simulink model "RHex1v3_Z_0v1b_PID"  (Simulink 7.9)
settings: Solver=ode23t  StartTime=0.0  StopTime=tp*3  MaxStep=0.005  RelTol=1e-3
values from neighbouring files (symbols this model uses):
  C = 100    [groundContact_init.m]
  Gvis = 0.01    [groundContact_init.m]
  K = x(5)    [PSO.m]    (also in PSO2_Kconst.m = 865; PSO3_PID.m = 525.4; bClockGen1v3_fin_acc.m = 1000; groundContact_init.m = 1000)
  kd = x(3)    [PSO3_PID.m]
  ki = x(2)    [PSO3_PID.m]
  kn = x(4)    [PSO3_PID.m]
  kp = x(1)    [PSO3_PID.m]
  m = 2    [PSO.m]    (also in PSO2_Kconst.m)
  nux = 1    [groundContact_init.m]
  nuy = 1    [groundContact_init.m]
  psziL = [psziL 360+psziL 720+psziL 1080+psziL]    [bClocGen1v3_fun.m]    (also in bClockGen1v3_fin_acc.m)
  psziR = [psziR 360+psziR 720+psziR 1080+psziR]    [bClocGen1v3_fun.m]    (also in bClockGen1v3_fin_acc.m)
  tp = x(1)    [PSO.m]    (also in PSO2_Kconst.m; PSO3_PID.m = 1.6; bClockGen1v3_fin_acc.m = 3)
undefined symbols (not defined in the file or in its folder): Body, deg, lab_rogz1v1, RHex1v3, RHex1v3_Z, RootPart, s
libraries: mblibv1 x64, Ervin x12, simulink x8
(part 1 of 2)
settings Model: Creator=Cloud  LastModifiedBy=Cloud
settings SimMechanicsCC: VisOnUpdateDiagram=on  VisDuringSimulation=on
settings ConfigurationSet: Description=SimMechanics 2G

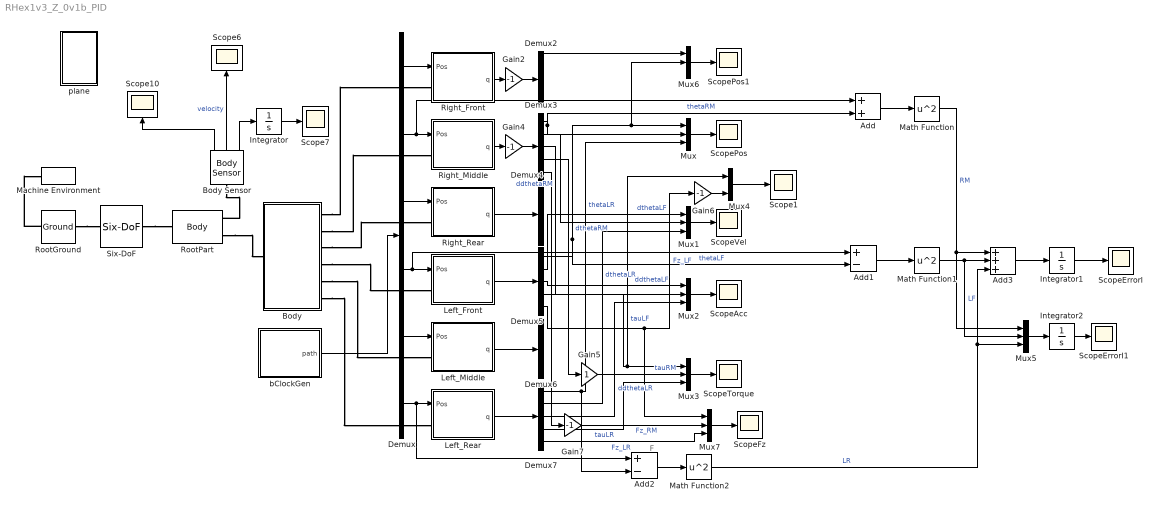
== system RHex1v3_Z_0v1b_PID ==
  note: F
  Add : Sum
  Add1 : Sum  Inputs=+-
  Add2 : Sum  Inputs=+-
  Add3 : Sum  Inputs=+++
  Body : Subsystem
  Body Sensor : mblibv1/Sensors &  Actuators/Body Sensor  UpdateFromCAD=off  PhysicalDomain=Mechanical  PortType=blob  Muxed=off  Pose=off  Angle=on  AngleUnits=deg  ArcVelocity=on  ArcVelocityUnits=deg/s  ArcAcceleration=off  ArcAccelerationUnits=deg/s^2  CoordPosition=on  CoordPositionUnits=mm  Velocity=on  VelocityUnits=m/s  Acceleration=off  AccelerationUnits=m/s^2  Quaternion=on  QuaternionDT=off  QuaternionDDT=off  QuaternionUnits=off  OutputVector=[1]  ActiveIO=on  Width=9  DialogClass=MechanicalSensorBlock  ReferenceFrame=Absolute (World)
  Demux : Demux  Outputs=6
  Demux{2..7} (6 alike) : Demux  Outputs=5
  Gain{2,4,6..7} (4 alike) : Gain  Gain=-1
  Gain5 : Gain
  Integrator : Integrator
  Integrator1 : Integrator
  Integrator2 : Integrator
  Left_Front : Subsystem
  Left_Middle : Subsystem
  Left_Rear : Subsystem
  Machine Environment : mblibv1/Bodies/Machine Environment  PortType=env  PhysicalDomain=Mechanical  DialogTemplateClass=MECH.MachineEnvironment  SyncWhenCopied=off  Gravity=[0 0 -9.81]  GravityUnits=m/s^2  GravityAsSignal=off  Dimensionality=Auto-detect  AnalysisType=Forward dynamics  LinearAssemblyTolerance=1e-3  LinearAssemblyToleranceUnits=m  AngularAssemblyTolerance=1e-3  AngularAssemblyToleranceUnits=rad  ConstraintSolverType=Stabilizing  ConstraintRelTolerance=1e-4  ConstraintAbsTolerance=1e-4  UseRobustSingularityHandling=off  RedundancyAnalysisToleranceType=Automatically select tolerance  RedundancyAnalysisTolerance=1e-14  StatePerturbationType=Fixed  PerturbationSize=1e-5  VisualizeMachine=on  BodyVisualizationType=Use model default body geometries  BodyColorSelMode=Use model default  DefaultBodyColor=[1 0 0]
  Math Function : Math  Operator=square  SaturateOnIntegerOverflow=on
  Math Function1 : Math  Operator=square  SaturateOnIntegerOverflow=on
  Math Function2 : Math  Operator=square  SaturateOnIntegerOverflow=on
  Mux{,1..3,5..7} (7 alike) : Mux  Inputs=3
  Mux4 : Mux  Inputs=2
  Right_Front : Subsystem
  Right_Middle : Subsystem
  Right_Rear : Subsystem
  RootGround : mblibv1/Bodies/Ground  UpdateFromCAD=on  PMImportedID=RootGround  LeftPortType=env  RightPortType=workingframe  PhysicalDomain=Mechanical  DialogClass=GroundBlock  CoordPosition=[-0.165584,-0.156961,0.0648014]  CoordPositionUnits=m  StateVectorMgrId=0  MachineId=[1 0]  ShowEnvPort=on
  RootPart : mblibv1/Bodies/Body  LConnTagsString=CS3  RConnTagsString=CG|CS2  UpdateFromCAD=on  PMImportedID=RHex1v3_Z/RootPart  DialogClass=MechanicalBodyBlock  Mass=0  MassUnits=kg  InertiaUnits=kg*m^2  Inertia=[0,0,0;0,0,0;0,0,0]  Shape=Cylinder  ShapeDims=[1 1]  ShapeUnits=m  ShapeUse=false  Density=1  DensityUnits=kg/m^3  DensityUse=false  GraphicsMode=MACHINE_DEFAULT  BodyColorSelMode=MACHINE_DEFAULT  BodyColor=[1 0 0]  AttachedToCS=CS1  CG=Right$CG$[-0.165584 -0.156961 0.0648014]$WORLD$WORLD$m$[1 0 0;0 1 0;0 0 1]$3x3 Transform$rad$WORLD$true$RHex1v3_Z/RootPart::CG(AUTOGEN)  WorkingFrames=Right$CS1$[0 0 0]$WORLD$WORLD$m$[1 0 0;0 1 0;0 0 1]$3x3 Transform$rad$WORLD$false$RHex1v3_Z/RootPart::CS1(AUTOGEN)#Right$CS2$[-0.165584 -0.154052 0.0672766]$WORLD$WORLD$m$[1 0 0;0 1 0;0 0 1]$3x3 Transform$rad$WORLD$true$Body^RHex1v3-1:-:RHex1v3_Z/RootPart::RHex1v3_Z/RootPart(AUTOGEN)#Left$CS3$[-0.165584 -0.156961 0.0648014]$WORLD$WORLD$m$[1 0 0;0 1 0;0 0 1]$3x3 Transform$rad$WORLD$true$RHex1v3_Z/RootPart:-:RootGround::RHex1v3_Z/RootPart(AUTOGEN)  CGPos=[-0.165584 -0.156961 0.0648014]  CGRot=[1 0 0;0 1 0;0 0 1]  CS0Pos=[]  CS0Rot=[]  CS1Pos=[0 0 0]  CS1Rot=[1 0 0;0 1 0;0 0 1]  CS2Pos=[-0.165584 -0.154052 0.0672766]  CS2Rot=[1 0 0;0 1 0;0 0 1]  CS3Pos=[-0.165584 -0.156961 0.0648014]  CS3Rot=[1 0 0;0 1 0;0 0 1]  CS4Pos=[]  CS4Rot=[]  CS5Pos=[]  CS5Rot=[]  CS6Pos=[]  CS6Rot=[]  CS7Pos=[]  CS7Rot=[]  CS8Pos=[]  CS8Rot=[]  CS9Pos=[]  CS9Rot=[]  CS10Pos=[]  CS10Rot=[]  CS11Pos=[]  CS11Rot=[]  CS12Pos=[]  CS12Rot=[]  CS13Pos=[]  CS13Rot=[]  CS14Pos=[]  CS14Rot=[]  CS15Pos=[]  CS15Rot=[]  CS16Pos=[]  CS16Rot=[]  CS17Pos=[]  CS17Rot=[]  CS18Pos=[]  CS18Rot=[]  CS19Pos=[]  CS19Rot=[]  CS20Pos=[]  CS20Rot=[]
  Scope{1,6..7,10} (4 alike) : Scope
      Scope1 settings: ShowLegends=on  YMin=-7  YMax=10  SaveName=ScopePos1
      Scope10 settings: ShowLegends=on  YMin=125  YMax=400  SaveName=ScopeBodyPos
      Scope6 settings: ShowLegends=on  YMin=-0.04  YMax=0.13  SaveName=ScopeBodyVel
      Scope7 settings: ShowLegends=on  YMin=-3.5  YMax=4  SaveName=ScopeBodyVel1
  ScopeAcc : Scope
      settings: ShowLegends=on  YMin=-3000  YMax=3000  SaveName=ScopeAcc
  ScopeErrorI : Scope
      settings: ShowLegends=on  YMin=0.004862  YMax=0.004884  SaveName=ScopeErrorI
  ScopeErrorI1 : Scope
      settings: ShowLegends=on  YMin=0  YMax=0.0017  SaveName=ScopeErrorI1
  ScopeFz : Scope
      settings: ShowLegends=on  YMin=-1.4  YMax=0.4  SaveName=ScopeFz
  ScopePos : Scope
      settings: ShowLegends=on  YMin=-200  YMax=200  SaveName=ScopePos
  ScopePos1 : Scope
      settings: ShowLegends=on  YMin=-200  YMax=200  SaveName=ScopePos2
  ScopeTorque : Scope
      settings: ShowLegends=on  YMin=-0.1  YMax=1.5  SaveName=ScopeTau
  ScopeVel : Scope
      settings: ShowLegends=on  YMin=-400  YMax=550  SaveName=ScopeVel
  Six-DoF : mblibv1/Joints/Six-DoF  LConnTagsString=__newl0  RConnTagsString=__newr0  UpdateFromCAD=off  NumSAPorts=0  CutJoint=off  MarkAsCut=off  Primitives=prismatic_prismatic  PrimitiveProps=P1$WORLD$[1 0 0]$prismatic#P2$WORLD$[0 1 0]$prismatic#P3$WORLD$[0 0 1]$prismatic#S$WORLD$[0 0 0]$spherical  DialogClass=JointBlock  P1Axis=[1 0 0]  P2Axis=[0 1 0]  P3Axis=[0 0 1]  SAxis=[0 0 0]
  bClockGen : Subsystem
  plane : Subsystem
  wires:
  Body Sensor/2 -> Scope6/1  "velocity"
  Body Sensor/1 -> Scope10/1
  Body Sensor/3 -> Integrator/1
  Integrator/1 -> Scope7/1
  Demux/1 -> Right_Front/1(Pos)
  Demux/2 -> Right_Middle/1(Pos), Add/1
  Demux/3 -> Right_Rear/1(Pos)
  Demux/4 -> Left_Front/1(Pos), Add1/1
  Demux/5 -> Left_Middle/1(Pos)
  Demux/6 -> Left_Rear/1(Pos), Add2/1
  bClockGen/1(path) -> Demux/1
  Right_Front/1(q) -> Gain2/1
  Right_Middle/1(q) -> Gain4/1
  Left_Middle/1(q) -> Demux6/1
  Gain4/1 -> Demux3/1
  Gain2/1 -> Demux2/1
  Right_Rear/1(q) -> Demux4/1
  Left_Front/1(q) -> Demux5/1
  Left_Rear/1(q) -> Demux7/1
  Demux3/5 -> Gain7/1
  Demux3/4 -> Gain5/1
  Mux/1 -> ScopePos/1
  Mux1/1 -> ScopeVel/1
  Mux2/1 -> ScopeAcc/1
  Mux3/1 -> ScopeTorque/1
  Demux5/1 -> Add1/2, Mux/1, Mux6/2  "thetaLF"
  Demux3/1 -> Mux/2, Add/2  "thetaRM"
  Demux7/1 -> Mux/3, Add2/2  "thetaLR"
  Demux3/2 -> Mux1/2  "dthetaRM"
  Demux5/2 -> Mux1/1  "dthetaLF"
  Demux7/2 -> Mux1/3  "dthetaLR"
  Demux3/3 -> Mux2/2  "ddthetaRM"
  Demux5/3 -> Mux2/1  "ddthetaLF"
  Demux7/3 -> Mux2/3  "ddthetaLR"
  Gain5/1 -> Mux3/2  "tauRM"
  Demux5/4 -> Mux3/1, Mux4/1  "tauLF"
  Demux7/4 -> Mux3/3  "tauLR"
  Mux4/1 -> Scope1/1
  Gain6/1 -> Mux4/2
  Demux5/5 -> Gain6/1, Mux7/1  "Fz_LF"
  Demux2/1 -> Mux6/1
  Mux6/1 -> ScopePos1/1
  Mux7/1 -> ScopeFz/1
  Gain7/1 -> Mux7/2  "Fz_RM"
  Demux7/5 -> Mux7/3  "Fz_LR"
  Add/1 -> Math Function/1
  Add1/1 -> Math Function1/1
  Add2/1 -> Math Function2/1
  Math Function/1 -> Add3/1, Mux5/1  "RM"
  Math Function1/1 -> Add3/2, Mux5/2  "LF"
  Math Function2/1 -> Add3/3, Mux5/3  "LR"
  Add3/1 -> Integrator1/1
  Mux5/1 -> Integrator2/1
  Integrator1/1 -> ScopeErrorI/1
  Integrator2/1 -> ScopeErrorI1/1
  connections:
  RootPart/RConn2 -- Body/LConn1
  Body/RConn4 -- Left_Front/LConn1
  Body/RConn3 -- Right_Rear/LConn1
  Body/RConn2 -- Right_Middle/LConn1
  Body/RConn1 -- Right_Front/LConn1
  Body/RConn6 -- Left_Rear/LConn1
  Body/RConn5 -- Left_Middle/LConn1
  RootGround/RConn1 -- Six-DoF/LConn1
  Six-DoF/RConn1 -- RootPart/LConn1
  RootGround/LConn1 -- Machine Environment/RConn1
  Body Sensor/LConn1 -- RootPart/RConn1

== system RHex1v3_Z_0v1b_PID/Body ==
  Body^RHex1v3-1 : mblibv1/Bodies/Body  LConnTagsString=CS2  RConnTagsString=CS3|CS4|CS5|CS6|CS7|CS8  UpdateFromCAD=on  PMImportedID=Body^RHex1v3-1  DialogClass=MechanicalBodyBlock  Mass=1.6487  MassUnits=kg  InertiaUnits=kg*m^2  Inertia=[0.0141689,9.04363e-10,1.498e-07;9.04363e-10,0.0230104,2.69394e-09;1.498e-07,2.69394e-09,0.00925721]  Shape=Cylinder  ShapeDims=[1 1]  ShapeUnits=m  ShapeUse=false  Density=1  DensityUnits=kg/m^3  DensityUse=false  GraphicsMode=GFXFILE  GraphicsFileName=RHex1v3_Z - Body^RHex1v3-1.STL  BodyColorSelMode=COLORPALETTE  BodyColor=[1;1;1]  AttachedToCS=CS1  CG=Right$CG$[-0.165584 -0.154052 0.0672766]$WORLD$WORLD$m$[-1 0 0;0 0 1;0 1 0]$3x3 Transform$rad$WORLD$false$Body^RHex1v3-1::CG(AUTOGEN)  WorkingFrames=Right$CS1$[-0.165584 -0.154051 0.0866787]$WORLD$WORLD$m$[-1 0 0;0 0 1;0 1 0]$3x3 Transform$rad$WORLD$false$Body^RHex1v3-1::CS1(AUTOGEN)#Left$CS2$[-0.165584 -0.154052 0.0672766]$WORLD$WORLD$m$[1 0 0;0 1 0;0 0 1]$3x3 Transform$rad$WORLD$true$Body^RHex1v3-1:-:RHex1v3_Z/RootPart::Body^RHex1v3-1(AUTOGEN)#Right$CS3$[-0.250584 -0.029051 0.0691787]$WORLD$WORLD$m$[1 0 0;0 1 0;0 0 1]$3x3 Transform$rad$WORLD$true$Body^RHex1v3-1:-:lab_rogz1v1-6::Body^RHex1v3-1(AUTOGEN)#Right$CS4$[-0.080584 -0.279051 0.0691787]$WORLD$WORLD$m$[1 0 0;0 1 0;0 0 1]$3x3 Transform$rad$WORLD$true$Body^RHex1v3-1:-:lab_rogz1v1-3::Body^RHex1v3-1(AUTOGEN)#Right$CS5$[-0.040584 -0.154051 0.0691787]$WORLD$WORLD$m$[1 0 0;0 1 0;0 0 1]$3x3 Transform$rad$WORLD$true$Body^RHex1v3-1:-:lab_rogz1v1-2::Body^RHex1v3-1(AUTOGEN)#Right$CS6$[-0.080584 -0.0290479 0.0691787]$WORLD$WORLD$m$[1 0 0;0 1 0;0 0 1]$3x3 Transform$rad$WORLD$true$Body^RHex1v3-1:-:lab_rogz1v1-1::Body^RHex1v3-1(AUTOGEN)#Right$CS7$[-0.250584 -0.279054 0.0691787]$WORLD$WORLD$m$[1 0 0;0 1 0;0 0 1]$3x3 Transform$rad$WORLD$true$Body^RHex1v3-1:-:lab_rogz1v1-4::Body^RHex1v3-1(AUTOGEN)#Right$CS8$[-0.290581 -0.154054 0.0691787]$WORLD$WORLD$m$[1 0 0;0 1 0;0 0 1]$3x3 Transform$rad$WORLD$true$Body^RHex1v3-1:-:lab_rogz1v1-5::Body^RHex1v3-1(AUTOGEN)  CGPos=[-0.165584 -0.154052 0.0672766]  CGRot=[-1 0 0;0 0 1;0 1 0]  CS0Pos=[]  CS0Rot=[]  CS1Pos=[-0.165584 -0.154051 0.0866787]  CS1Rot=[-1 0 0;0 0 1;0 1 0]  CS2Pos=[-0.165584 -0.154052 0.0672766]  CS2Rot=[1 0 0;0 1 0;0 0 1]  CS3Pos=[-0.250584 -0.029051 0.0691787]  CS3Rot=[1 0 0;0 1 0;0 0 1]  CS4Pos=[-0.080584 -0.279051 0.0691787]  CS4Rot=[1 0 0;0 1 0;0 0 1]  CS5Pos=[-0.040584 -0.154051 0.0691787]  CS5Rot=[1 0 0;0 1 0;0 0 1]  CS6Pos=[-0.080584 -0.0290479 0.0691787]  CS6Rot=[1 0 0;0 1 0;0 0 1]  CS7Pos=[-0.250584 -0.279054 0.0691787]  CS7Rot=[1 0 0;0 1 0;0 0 1]  CS8Pos=[-0.290581 -0.154054 0.0691787]  CS8Rot=[1 0 0;0 1 0;0 0 1]  CS9Pos=[]  CS9Rot=[]  CS10Pos=[]  CS10Rot=[]  CS11Pos=[]  CS11Rot=[]  CS12Pos=[]  CS12Rot=[]  CS13Pos=[]  CS13Rot=[]  CS14Pos=[]  CS14Rot=[]  CS15Pos=[]  CS15Rot=[]  CS16Pos=[]  CS16Rot=[]  CS17Pos=[]  CS17Rot=[]  CS18Pos=[]  CS18Rot=[]  CS19Pos=[]  CS19Rot=[]  CS20Pos=[]  CS20Rot=[]
  Weld : mblibv1/Joints/Weld  LConnTagsString=__newl0  RConnTagsString=__newr0  UpdateFromCAD=on  PMImportedID=Body^RHex1v3-1:-:RHex1v3_Z/RootPart  NumSAPorts=0  CutJoint=off  MarkAsCut=off  Primitives=weld  PrimitiveProps=W$WORLD$[0.57735,0.57735,0.57735]$weld  DialogClass=JointBlock  WAxis=[0.57735,0.57735,0.57735]
  RF : PMIOPort  Port=1  Side=Right
  RM : PMIOPort  Port=2  Side=Right
  RR : PMIOPort  Port=3  Side=Right
  LF : PMIOPort  Port=4  Side=Right
  LM : PMIOPort  Port=5  Side=Right
  LR : PMIOPort  Port=6  Side=Right
  Root : PMIOPort  Port=7  Side=Left
  connections:
  Weld/RConn1 -- Body^RHex1v3-1/LConn1
  LF/RConn1 -- Body^RHex1v3-1/RConn1
  RR/RConn1 -- Body^RHex1v3-1/RConn2
  RM/RConn1 -- Body^RHex1v3-1/RConn3
  RF/RConn1 -- Body^RHex1v3-1/RConn4
  Root/RConn1 -- Weld/LConn1
  LR/RConn1 -- Body^RHex1v3-1/RConn5
  LM/RConn1 -- Body^RHex1v3-1/RConn6

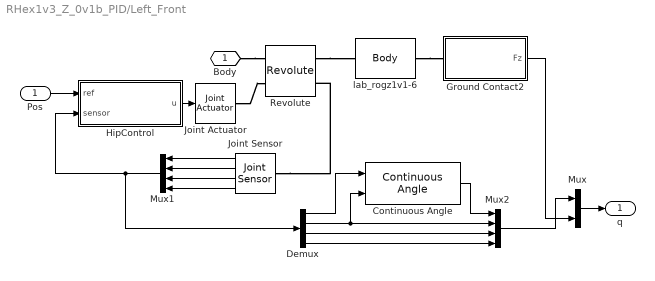
== system RHex1v3_Z_0v1b_PID/Left_Front ==
  Pos : Inport
  Continuous Angle : mblibv1/Utilities/Continuous Angle  rad=deg  rads=deg/s
  Demux : Demux
  Ground Contact2 : Subsystem  AncestorBlock=Ervin/Ground Contact
  HipControl : Subsystem
  Joint Actuator : mblibv1/Sensors &  Actuators/Joint Actuator  UpdateFromCAD=off  PhysicalDomain=Mechanical  PortType=blob  ActuationStyle=Force  AngleUnits=deg  ArcVelocityUnits=deg/s  ArcAccelerationUnits=deg/s^2  CoordPositionUnits=m  VelocityUnits=m/s  AccelerationUnits=m/s^2  ForceUnits=N  TorqueUnits=N-m  ActiveIO=on  Width=1  DialogClass=MechanicalActuatorBlock  Primitive=R1  ReferenceFrame=Absolute (World)
  Joint Sensor : mblibv1/Sensors &  Actuators/Joint Sensor  UpdateFromCAD=off  PhysicalDomain=Mechanical  PortType=blob  Muxed=off  Pose=off  Angle=on  AngleUnits=deg  ArcVelocity=on  ArcVelocityUnits=deg/s  ArcAcceleration=on  ArcAccelerationUnits=deg/s^2  CoordPosition=on  CoordPositionUnits=m  Velocity=off  VelocityUnits=m/s  Acceleration=off  AccelerationUnits=m/s^2  Quaternion=on  QuaternionDT=off  QuaternionDDT=off  QuaternionUnits=off  OutputVector=[1]  ActiveIO=on  Width=4  DialogClass=MechanicalSensorBlock  Primitive=R1  Force=off  ForceUnits=N  Torque=on  TorqueUnits=N*m  ReferenceFrame=Absolute (World)  ReactionSensedSide=Base  ReactionReferenceFrame=Absolute (World)  ReactionForce=off  ReactionForceUnits=N  ReactionMoment=off  ReactionMomentUnits=N*m
  Mux : Mux  Inputs=2
  Mux1 : Mux
  Mux2 : Mux
  Revolute : mblibv1/Joints/Revolute  LConnTagsString=__newl0|SA1  RConnTagsString=__newr0|SA1  UpdateFromCAD=on  PMImportedID=Body^RHex1v3-1:-:lab_rogz1v1-6  NumSAPorts=2  CutJoint=off  MarkAsCut=off  Primitives=prismatic  PrimitiveProps=R1$World$[-1,0,0]$revolute  DialogClass=JointBlock  R1Axis=[-1,0,0]
  lab_rogz1v1-6 : mblibv1/Bodies/Body  LConnTagsString=CS2  RConnTagsString=CS3  UpdateFromCAD=on  PMImportedID=lab_rogz1v1-6  DialogClass=MechanicalBodyBlock  Mass=0.0510405  MassUnits=kg  InertiaUnits=kg*m^2  Inertia=[7.74224e-05,-1.05103e-11,2.05656e-12;-1.05103e-11,2.14517e-05,-6.14042e-06;2.05656e-12,-6.14042e-06,6.37147e-05]  Shape=Cylinder  ShapeDims=[1 1]  ShapeUnits=m  ShapeUse=false  Density=1  DensityUnits=kg/m^3  DensityUse=false  GraphicsMode=GFXFILE  GraphicsFileName=RHex1v3_Z - lab_rogz1v1-6.STL  BodyColorSelMode=COLORPALETTE  BodyColor=[0 0.49804 0]  AttachedToCS=CS1  CG=Right$CG$[-0.277584 -0.0476207 0.0516204]$WORLD$WORLD$m$[-1 0 0;0 0 1;0 1 0]$3x3 Transform$rad$WORLD$false$lab_rogz1v1-6::CG(AUTOGEN)  WorkingFrames=Right$CS1$[-0.262584 -0.014051 0.00353831]$WORLD$WORLD$m$[-1 0 0;0 0 1;0 1 0]$3x3 Transform$rad$WORLD$false$lab_rogz1v1-6::CS1(AUTOGEN)#Left$CS2$[-0.250584 -0.029051 0.0691787]$WORLD$WORLD$m$[1 0 0;0 1 0;0 0 1]$3x3 Transform$rad$WORLD$true$Body^RHex1v3-1:-:lab_rogz1v1-6::lab_rogz1v1-6(AUTOGEN)#Right$CS3$[-0.277584 -0.029051 -0.0258213]$WORLD$WORLD$m$[1 0 0;0 1 0;0 0 1]$3x3 Transform$rad$WORLD$true$dummy-4:-:lab_rogz1v1-6::lab_rogz1v1-6(AUTOGEN)  CGPos=[-0.277584 -0.0476207 0.0516204]  CGRot=[-1 0 0;0 0 1;0 1 0]  CS0Pos=[]  CS0Rot=[]  CS1Pos=[-0.262584 -0.014051 0.00353831]  CS1Rot=[-1 0 0;0 0 1;0 1 0]  CS2Pos=[-0.250584 -0.029051 0.0691787]  CS2Rot=[1 0 0;0 1 0;0 0 1]  CS3Pos=[-0.277584 -0.029051 -0.0258213]  CS3Rot=[1 0 0;0 1 0;0 0 1]  CS4Pos=[]  CS4Rot=[]  CS5Pos=[]  CS5Rot=[]  CS6Pos=[]  CS6Rot=[]  CS7Pos=[]  CS7Rot=[]  CS8Pos=[]  CS8Rot=[]  CS9Pos=[]  CS9Rot=[]  CS10Pos=[]  CS10Rot=[]  CS11Pos=[]  CS11Rot=[]  CS12Pos=[]  CS12Rot=[]  CS13Pos=[]  CS13Rot=[]  CS14Pos=[]  CS14Rot=[]  CS15Pos=[]  CS15Rot=[]  CS16Pos=[]  CS16Rot=[]  CS17Pos=[]  CS17Rot=[]  CS18Pos=[]  CS18Rot=[]  CS19Pos=[]  CS19Rot=[]  CS20Pos=[]  CS20Rot=[]
  Body : PMIOPort  Port=1  Side=Left
  q : Outport
  wires:
  Ground Contact2/1(Fz) -> Mux/2
  HipControl/1(u) -> Joint Actuator/1
  Mux1/1 -> HipControl/2(sensor), Demux/1
  Joint Sensor/1 -> Mux1/1
  Joint Sensor/2 -> Mux1/2
  Joint Sensor/3 -> Mux1/3
  Joint Sensor/4 -> Mux1/4
  Pos/1 -> HipControl/1(ref)
  Mux/1 -> q/1
  Demux/1 -> Continuous Angle/1
  Demux/2 -> Continuous Angle/2, Mux2/2
  Continuous Angle/1 -> Mux2/1
  Demux/3 -> Mux2/3
  Demux/4 -> Mux2/4
  Mux2/1 -> Mux/1
  connections:
  lab_rogz1v1-6/RConn1 -- Ground Contact2/LConn1
  Joint Actuator/RConn1 -- Revolute/LConn2
  Joint Sensor/LConn1 -- Revolute/RConn2
  Revolute/RConn1 -- lab_rogz1v1-6/LConn1
  Body/RConn1 -- Revolute/LConn1

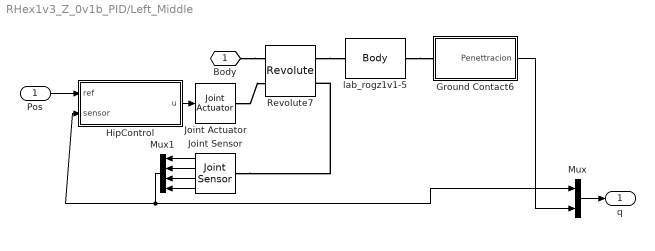
== system RHex1v3_Z_0v1b_PID/Left_Middle ==
  Pos : Inport
  Ground Contact6 : Subsystem  AncestorBlock=Ervin/Ground Contact
  HipControl : Subsystem
  Joint Actuator : mblibv1/Sensors &  Actuators/Joint Actuator  UpdateFromCAD=off  PhysicalDomain=Mechanical  PortType=blob  ActuationStyle=Force  AngleUnits=deg  ArcVelocityUnits=deg/s  ArcAccelerationUnits=deg/s^2  CoordPositionUnits=m  VelocityUnits=m/s  AccelerationUnits=m/s^2  ForceUnits=N  TorqueUnits=N-m  ActiveIO=on  Width=1  DialogClass=MechanicalActuatorBlock  Primitive=R1  ReferenceFrame=Absolute (World)
  Joint Sensor : mblibv1/Sensors &  Actuators/Joint Sensor  UpdateFromCAD=off  PhysicalDomain=Mechanical  PortType=blob  Muxed=off  Pose=off  Angle=on  AngleUnits=deg  ArcVelocity=on  ArcVelocityUnits=deg/s  ArcAcceleration=on  ArcAccelerationUnits=deg/s^2  CoordPosition=on  CoordPositionUnits=m  Velocity=off  VelocityUnits=m/s  Acceleration=off  AccelerationUnits=m/s^2  Quaternion=on  QuaternionDT=off  QuaternionDDT=off  QuaternionUnits=off  OutputVector=[1]  ActiveIO=on  Width=4  DialogClass=MechanicalSensorBlock  Primitive=R1  Force=off  ForceUnits=N  Torque=on  TorqueUnits=N*m  ReferenceFrame=Absolute (World)  ReactionSensedSide=Base  ReactionReferenceFrame=Absolute (World)  ReactionForce=off  ReactionForceUnits=N  ReactionMoment=off  ReactionMomentUnits=N*m
  Mux : Mux  Inputs=2
  Mux1 : Mux
  Revolute7 : mblibv1/Joints/Revolute  LConnTagsString=__newl0|SA1  RConnTagsString=__newr0|SA1  UpdateFromCAD=on  PMImportedID=Body^RHex1v3-1:-:lab_rogz1v1-5  NumSAPorts=2  CutJoint=off  MarkAsCut=off  Primitives=prismatic  PrimitiveProps=R1$World$[-1,0,0]$revolute  DialogClass=JointBlock  R1Axis=[-1,0,0]
  lab_rogz1v1-5 : mblibv1/Bodies/Body  LConnTagsString=CS2  RConnTagsString=CS3  UpdateFromCAD=on  PMImportedID=lab_rogz1v1-5  DialogClass=MechanicalBodyBlock  Mass=0.0510405  MassUnits=kg  InertiaUnits=kg*m^2  Inertia=[7.74224e-05,-1.05103e-11,2.05656e-12;-1.05103e-11,2.14517e-05,-6.14042e-06;2.05656e-12,-6.14042e-06,6.37147e-05]  Shape=Cylinder  ShapeDims=[1 1]  ShapeUnits=m  ShapeUse=false  Density=1  DensityUnits=kg/m^3  DensityUse=false  GraphicsMode=GFXFILE  GraphicsFileName=RHex1v3_Z - lab_rogz1v1-5.STL  BodyColorSelMode=COLORPALETTE  BodyColor=[0;0.498039;0]  AttachedToCS=CS1  CG=Right$CG$[-0.317581 -0.172624 0.0516204]$WORLD$WORLD$m$[-1 0 0;0 0 1;0 1 0]$3x3 Transform$rad$WORLD$false$lab_rogz1v1-5::CG(AUTOGEN)  WorkingFrames=Right$CS1$[-0.302581 -0.139054 0.00353831]$WORLD$WORLD$m$[-1 0 0;0 0 1;0 1 0]$3x3 Transform$rad$WORLD$false$lab_rogz1v1-5::CS1(AUTOGEN)#Left$CS2$[-0.290581 -0.154054 0.0691787]$WORLD$WORLD$m$[1 0 0;0 1 0;0 0 1]$3x3 Transform$rad$WORLD$true$Body^RHex1v3-1:-:lab_rogz1v1-5::lab_rogz1v1-5(AUTOGEN)#Right$CS3$[-0.317581 -0.154054 -0.0258213]$WORLD$WORLD$m$[1 0 0;0 1 0;0 0 1]$3x3 Transform$rad$WORLD$true$dummy-5:-:lab_rogz1v1-5::lab_rogz1v1-5(AUTOGEN)  CGPos=[-0.317581 -0.172624 0.0516204]  CGRot=[-1 0 0;0 0 1;0 1 0]  CS0Pos=[]  CS0Rot=[]  CS1Pos=[-0.302581 -0.139054 0.00353831]  CS1Rot=[-1 0 0;0 0 1;0 1 0]  CS2Pos=[-0.290581 -0.154054 0.0691787]  CS2Rot=[1 0 0;0 1 0;0 0 1]  CS3Pos=[-0.317581 -0.154054 -0.0258213]  CS3Rot=[1 0 0;0 1 0;0 0 1]  CS4Pos=[]  CS4Rot=[]  CS5Pos=[]  CS5Rot=[]  CS6Pos=[]  CS6Rot=[]  CS7Pos=[]  CS7Rot=[]  CS8Pos=[]  CS8Rot=[]  CS9Pos=[]  CS9Rot=[]  CS10Pos=[]  CS10Rot=[]  CS11Pos=[]  CS11Rot=[]  CS12Pos=[]  CS12Rot=[]  CS13Pos=[]  CS13Rot=[]  CS14Pos=[]  CS14Rot=[]  CS15Pos=[]  CS15Rot=[]  CS16Pos=[]  CS16Rot=[]  CS17Pos=[]  CS17Rot=[]  CS18Pos=[]  CS18Rot=[]  CS19Pos=[]  CS19Rot=[]  CS20Pos=[]  CS20Rot=[]
  Body : PMIOPort  Port=1  Side=Left
  q : Outport
  wires:
  Pos/1 -> HipControl/1(ref)
  Ground Contact6/1(Penettracion) -> Mux/2
  HipControl/1(u) -> Joint Actuator/1
  Mux1/1 -> Mux/1, HipControl/2(sensor)
  Joint Sensor/1 -> Mux1/1
  Joint Sensor/2 -> Mux1/2
  Joint Sensor/3 -> Mux1/3
  Joint Sensor/4 -> Mux1/4
  Mux/1 -> q/1
  connections:
  lab_rogz1v1-5/RConn1 -- Ground Contact6/LConn1
  Joint Actuator/RConn1 -- Revolute7/LConn2
  Joint Sensor/LConn1 -- Revolute7/RConn2
  Revolute7/RConn1 -- lab_rogz1v1-5/LConn1
  Body/RConn1 -- Revolute7/LConn1

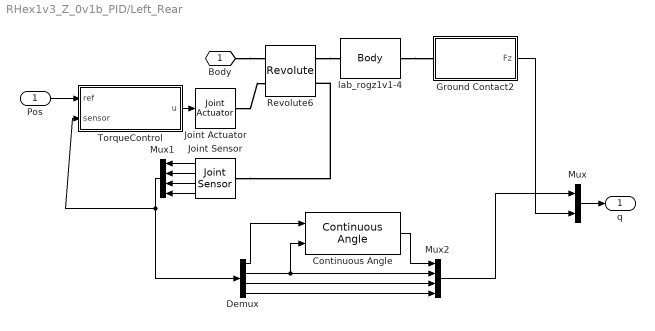
== system RHex1v3_Z_0v1b_PID/Left_Rear ==
  Pos : Inport
  Continuous Angle : mblibv1/Utilities/Continuous Angle  rad=deg  rads=deg/s
  Demux : Demux
  Ground Contact2 : Subsystem  AncestorBlock=Ervin/Ground Contact
  Joint Actuator : mblibv1/Sensors &  Actuators/Joint Actuator  UpdateFromCAD=off  PhysicalDomain=Mechanical  PortType=blob  ActuationStyle=Force  AngleUnits=deg  ArcVelocityUnits=deg/s  ArcAccelerationUnits=deg/s^2  CoordPositionUnits=m  VelocityUnits=m/s  AccelerationUnits=m/s^2  ForceUnits=N  TorqueUnits=N-m  ActiveIO=on  Width=1  DialogClass=MechanicalActuatorBlock  Primitive=R1  ReferenceFrame=Absolute (World)
  Joint Sensor : mblibv1/Sensors &  Actuators/Joint Sensor  UpdateFromCAD=off  PhysicalDomain=Mechanical  PortType=blob  Muxed=off  Pose=off  Angle=on  AngleUnits=deg  ArcVelocity=on  ArcVelocityUnits=deg/s  ArcAcceleration=on  ArcAccelerationUnits=deg/s^2  CoordPosition=on  CoordPositionUnits=m  Velocity=off  VelocityUnits=m/s  Acceleration=off  AccelerationUnits=m/s^2  Quaternion=on  QuaternionDT=off  QuaternionDDT=off  QuaternionUnits=off  OutputVector=[1]  ActiveIO=on  Width=4  DialogClass=MechanicalSensorBlock  Primitive=R1  Force=off  ForceUnits=N  Torque=on  TorqueUnits=N*m  ReferenceFrame=Absolute (World)  ReactionSensedSide=Base  ReactionReferenceFrame=Absolute (World)  ReactionForce=off  ReactionForceUnits=N  ReactionMoment=off  ReactionMomentUnits=N*m
  Mux : Mux  Inputs=2
  Mux1 : Mux
  Mux2 : Mux
  Revolute6 : mblibv1/Joints/Revolute  LConnTagsString=__newl0|SA1  RConnTagsString=__newr0|SA1  UpdateFromCAD=on  PMImportedID=Body^RHex1v3-1:-:lab_rogz1v1-4  NumSAPorts=2  CutJoint=off  MarkAsCut=off  Primitives=prismatic  PrimitiveProps=R1$World$[-1,0,0]$revolute  DialogClass=JointBlock  R1Axis=[-1,0,0]
  TorqueControl : Subsystem
  lab_rogz1v1-4 : mblibv1/Bodies/Body  LConnTagsString=CS2  RConnTagsString=CS3  UpdateFromCAD=on  PMImportedID=lab_rogz1v1-4  DialogClass=MechanicalBodyBlock  Mass=0.0510405  MassUnits=kg  InertiaUnits=kg*m^2  Inertia=[7.74224e-05,-1.05103e-11,2.05656e-12;-1.05103e-11,2.14517e-05,-6.14042e-06;2.05656e-12,-6.14042e-06,6.37147e-05]  Shape=Cylinder  ShapeDims=[1 1]  ShapeUnits=m  ShapeUse=false  Density=1  DensityUnits=kg/m^3  DensityUse=false  GraphicsMode=GFXFILE  GraphicsFileName=RHex1v3_Z - lab_rogz1v1-4.STL  BodyColorSelMode=COLORPALETTE  BodyColor=[0;0.498039;0]  AttachedToCS=CS1  CG=Right$CG$[-0.277584 -0.297624 0.0516204]$WORLD$WORLD$m$[-1 0 0;0 0 1;0 1 0]$3x3 Transform$rad$WORLD$false$lab_rogz1v1-4::CG(AUTOGEN)  WorkingFrames=Right$CS1$[-0.262584 -0.264054 0.00353831]$WORLD$WORLD$m$[-1 0 0;0 0 1;0 1 0]$3x3 Transform$rad$WORLD$false$lab_rogz1v1-4::CS1(AUTOGEN)#Left$CS2$[-0.250584 -0.279054 0.0691787]$WORLD$WORLD$m$[1 0 0;0 1 0;0 0 1]$3x3 Transform$rad$WORLD$true$Body^RHex1v3-1:-:lab_rogz1v1-4::lab_rogz1v1-4(AUTOGEN)#Right$CS3$[-0.277584 -0.279054 -0.0258213]$WORLD$WORLD$m$[1 0 0;0 1 0;0 0 1]$3x3 Transform$rad$WORLD$true$dummy-6:-:lab_rogz1v1-4::lab_rogz1v1-4(AUTOGEN)  CGPos=[-0.277584 -0.297624 0.0516204]  CGRot=[-1 0 0;0 0 1;0 1 0]  CS0Pos=[]  CS0Rot=[]  CS1Pos=[-0.262584 -0.264054 0.00353831]  CS1Rot=[-1 0 0;0 0 1;0 1 0]  CS2Pos=[-0.250584 -0.279054 0.0691787]  CS2Rot=[1 0 0;0 1 0;0 0 1]  CS3Pos=[-0.277584 -0.279054 -0.0258213]  CS3Rot=[1 0 0;0 1 0;0 0 1]  CS4Pos=[]  CS4Rot=[]  CS5Pos=[]  CS5Rot=[]  CS6Pos=[]  CS6Rot=[]  CS7Pos=[]  CS7Rot=[]  CS8Pos=[]  CS8Rot=[]  CS9Pos=[]  CS9Rot=[]  CS10Pos=[]  CS10Rot=[]  CS11Pos=[]  CS11Rot=[]  CS12Pos=[]  CS12Rot=[]  CS13Pos=[]  CS13Rot=[]  CS14Pos=[]  CS14Rot=[]  CS15Pos=[]  CS15Rot=[]  CS16Pos=[]  CS16Rot=[]  CS17Pos=[]  CS17Rot=[]  CS18Pos=[]  CS18Rot=[]  CS19Pos=[]  CS19Rot=[]  CS20Pos=[]  CS20Rot=[]
  Body : PMIOPort  Port=1  Side=Left
  q : Outport
  wires:
  Ground Contact2/1(Fz) -> Mux/2
  TorqueControl/1(u) -> Joint Actuator/1
  Mux1/1 -> TorqueControl/2(sensor), Demux/1
  Joint Sensor/1 -> Mux1/1
  Joint Sensor/2 -> Mux1/2
  Joint Sensor/3 -> Mux1/3
  Joint Sensor/4 -> Mux1/4
  Pos/1 -> TorqueControl/1(ref)
  Mux/1 -> q/1
  Demux/1 -> Continuous Angle/1
  Demux/2 -> Continuous Angle/2, Mux2/2
  Continuous Angle/1 -> Mux2/1
  Demux/3 -> Mux2/3
  Demux/4 -> Mux2/4
  Mux2/1 -> Mux/1
  connections:
  lab_rogz1v1-4/RConn1 -- Ground Contact2/LConn1
  Joint Actuator/RConn1 -- Revolute6/LConn2
  Joint Sensor/LConn1 -- Revolute6/RConn2
  Revolute6/RConn1 -- lab_rogz1v1-4/LConn1
  Body/RConn1 -- Revolute6/LConn1

== system RHex1v3_Z_0v1b_PID/Right_Front ==
  Pos : Inport
  Ground Contact4 : Subsystem  AncestorBlock=Ervin/Ground Contact
  HipControl : Subsystem
  Joint Actuator1 : mblibv1/Sensors &  Actuators/Joint Actuator  UpdateFromCAD=off  PhysicalDomain=Mechanical  PortType=blob  ActuationStyle=Force  AngleUnits=deg  ArcVelocityUnits=deg/s  ArcAccelerationUnits=deg/s^2  CoordPositionUnits=m  VelocityUnits=m/s  AccelerationUnits=m/s^2  ForceUnits=N  TorqueUnits=N-m  ActiveIO=on  Width=1  DialogClass=MechanicalActuatorBlock  Primitive=R1  ReferenceFrame=Absolute (World)
  Joint Sensor1 : mblibv1/Sensors &  Actuators/Joint Sensor  UpdateFromCAD=off  PhysicalDomain=Mechanical  PortType=blob  Muxed=off  Pose=off  Angle=on  AngleUnits=deg  ArcVelocity=on  ArcVelocityUnits=deg/s  ArcAcceleration=on  ArcAccelerationUnits=deg/s^2  CoordPosition=on  CoordPositionUnits=m  Velocity=off  VelocityUnits=m/s  Acceleration=off  AccelerationUnits=m/s^2  Quaternion=on  QuaternionDT=off  QuaternionDDT=off  QuaternionUnits=off  OutputVector=[1]  ActiveIO=on  Width=4  DialogClass=MechanicalSensorBlock  Primitive=R1  Force=off  ForceUnits=N  Torque=on  TorqueUnits=N*m  ReferenceFrame=Absolute (World)  ReactionSensedSide=Base  ReactionReferenceFrame=Absolute (World)  ReactionForce=off  ReactionForceUnits=N  ReactionMoment=off  ReactionMomentUnits=N*m
  Mux2 : Mux  Inputs=2
  Mux3 : Mux
  Revolute5 : mblibv1/Joints/Revolute  LConnTagsString=__newl0|SA1  RConnTagsString=__newr0|SA1  UpdateFromCAD=on  PMImportedID=Body^RHex1v3-1:-:lab_rogz1v1-1  NumSAPorts=2  CutJoint=off  MarkAsCut=off  Primitives=prismatic  PrimitiveProps=R1$World$[1,0,0]$revolute  DialogClass=JointBlock  R1Axis=[1,0,0]
  lab_rogz1v1-1 : mblibv1/Bodies/Body  LConnTagsString=CS2  RConnTagsString=CS3  UpdateFromCAD=on  PMImportedID=lab_rogz1v1-1  DialogClass=MechanicalBodyBlock  Mass=0.0510405  MassUnits=kg  InertiaUnits=kg*m^2  Inertia=[7.74224e-05,-1.05103e-11,2.05656e-12;-1.05103e-11,2.14517e-05,-6.14042e-06;2.05656e-12,-6.14042e-06,6.37147e-05]  Shape=Cylinder  ShapeDims=[1 1]  ShapeUnits=m  ShapeUse=false  Density=1  DensityUnits=kg/m^3  DensityUse=false  GraphicsMode=GFXFILE  GraphicsFileName=RHex1v3_Z - lab_rogz1v1-1.STL  BodyColorSelMode=COLORPALETTE  BodyColor=[0;0.498039;0]  AttachedToCS=CS1  CG=Right$CG$[-0.053584 -0.0476176 0.0516204]$WORLD$WORLD$m$[-1 0 0;0 0 1;0 1 0]$3x3 Transform$rad$WORLD$false$lab_rogz1v1-1::CG(AUTOGEN)  WorkingFrames=Right$CS1$[-0.038584 -0.0140479 0.00353831]$WORLD$WORLD$m$[-1 0 0;0 0 1;0 1 0]$3x3 Transform$rad$WORLD$false$lab_rogz1v1-1::CS1(AUTOGEN)#Left$CS2$[-0.080584 -0.0290479 0.0691787]$WORLD$WORLD$m$[1 0 0;0 1 0;0 0 1]$3x3 Transform$rad$WORLD$true$Body^RHex1v3-1:-:lab_rogz1v1-1::lab_rogz1v1-1(AUTOGEN)#Right$CS3$[-0.053584 -0.0290479 -0.0258213]$WORLD$WORLD$m$[1 0 0;0 1 0;0 0 1]$3x3 Transform$rad$WORLD$true$dummy-1:-:lab_rogz1v1-1::lab_rogz1v1-1(AUTOGEN)  CGPos=[-0.053584 -0.0476176 0.0516204]  CGRot=[-1 0 0;0 0 1;0 1 0]  CS0Pos=[]  CS0Rot=[]  CS1Pos=[-0.038584 -0.0140479 0.00353831]  CS1Rot=[-1 0 0;0 0 1;0 1 0]  CS2Pos=[-0.080584 -0.0290479 0.0691787]  CS2Rot=[1 0 0;0 1 0;0 0 1]  CS3Pos=[-0.053584 -0.0290479 -0.0258213]  CS3Rot=[1 0 0;0 1 0;0 0 1]  CS4Pos=[]  CS4Rot=[]  CS5Pos=[]  CS5Rot=[]  CS6Pos=[]  CS6Rot=[]  CS7Pos=[]  CS7Rot=[]  CS8Pos=[]  CS8Rot=[]  CS9Pos=[]  CS9Rot=[]  CS10Pos=[]  CS10Rot=[]  CS11Pos=[]  CS11Rot=[]  CS12Pos=[]  CS12Rot=[]  CS13Pos=[]  CS13Rot=[]  CS14Pos=[]  CS14Rot=[]  CS15Pos=[]  CS15Rot=[]  CS16Pos=[]  CS16Rot=[]  CS17Pos=[]  CS17Rot=[]  CS18Pos=[]  CS18Rot=[]  CS19Pos=[]  CS19Rot=[]  CS20Pos=[]  CS20Rot=[]
  Body : PMIOPort  Port=1  Side=Left
  q : Outport
  wires:
  Ground Contact4/1(Penettracion) -> Mux2/2
  HipControl/1(u) -> Joint Actuator1/1
  Mux3/1 -> Mux2/1, HipControl/2(sensor)
  Joint Sensor1/1 -> Mux3/1
  Joint Sensor1/2 -> Mux3/2
  Joint Sensor1/3 -> Mux3/3
  Joint Sensor1/4 -> Mux3/4
  Pos/1 -> HipControl/1(ref)
  Mux2/1 -> q/1
  connections:
  lab_rogz1v1-1/RConn1 -- Ground Contact4/LConn1
  Joint Actuator1/RConn1 -- Revolute5/LConn2
  Joint Sensor1/LConn1 -- Revolute5/RConn2
  Revolute5/RConn1 -- lab_rogz1v1-1/LConn1
  Body/RConn1 -- Revolute5/LConn1

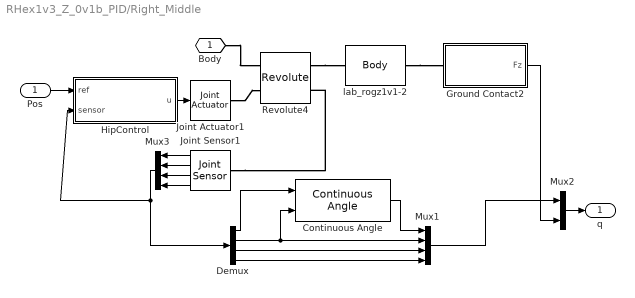
== system RHex1v3_Z_0v1b_PID/Right_Middle ==
  Pos : Inport
  Continuous Angle : mblibv1/Utilities/Continuous Angle  rad=deg  rads=deg/s
  Demux : Demux
  Ground Contact2 : Subsystem  AncestorBlock=Ervin/Ground Contact
  HipControl : Subsystem
  Joint Actuator1 : mblibv1/Sensors &  Actuators/Joint Actuator  UpdateFromCAD=off  PhysicalDomain=Mechanical  PortType=blob  ActuationStyle=Force  AngleUnits=deg  ArcVelocityUnits=deg/s  ArcAccelerationUnits=deg/s^2  CoordPositionUnits=m  VelocityUnits=m/s  AccelerationUnits=m/s^2  ForceUnits=N  TorqueUnits=N-m  ActiveIO=on  Width=1  DialogClass=MechanicalActuatorBlock  Primitive=R1  ReferenceFrame=Absolute (World)
  Joint Sensor1 : mblibv1/Sensors &  Actuators/Joint Sensor  UpdateFromCAD=off  PhysicalDomain=Mechanical  PortType=blob  Muxed=off  Pose=off  Angle=on  AngleUnits=deg  ArcVelocity=on  ArcVelocityUnits=deg/s  ArcAcceleration=on  ArcAccelerationUnits=deg/s^2  CoordPosition=on  CoordPositionUnits=m  Velocity=off  VelocityUnits=m/s  Acceleration=off  AccelerationUnits=m/s^2  Quaternion=on  QuaternionDT=off  QuaternionDDT=off  QuaternionUnits=off  OutputVector=[1]  ActiveIO=on  Width=4  DialogClass=MechanicalSensorBlock  Primitive=R1  Force=off  ForceUnits=N  Torque=on  TorqueUnits=N*m  ReferenceFrame=Absolute (World)  ReactionSensedSide=Base  ReactionReferenceFrame=Absolute (World)  ReactionForce=off  ReactionForceUnits=N  ReactionMoment=off  ReactionMomentUnits=N*m
  Mux1 : Mux
  Mux2 : Mux  Inputs=2
  Mux3 : Mux
  Revolute4 : mblibv1/Joints/Revolute  LConnTagsString=__newl0|SA1  RConnTagsString=__newr0|SA1  UpdateFromCAD=on  PMImportedID=Body^RHex1v3-1:-:lab_rogz1v1-2  NumSAPorts=2  CutJoint=off  MarkAsCut=off  Primitives=prismatic  PrimitiveProps=R1$World$[1,0,0]$revolute  DialogClass=JointBlock  R1Axis=[1,0,0]
  lab_rogz1v1-2 : mblibv1/Bodies/Body  LConnTagsString=CS2  RConnTagsString=CS3  UpdateFromCAD=on  PMImportedID=lab_rogz1v1-2  DialogClass=MechanicalBodyBlock  Mass=0.0510405  MassUnits=kg  InertiaUnits=kg*m^2  Inertia=[7.74224e-05,-1.05103e-11,2.05656e-12;-1.05103e-11,2.14517e-05,-6.14042e-06;2.05656e-12,-6.14042e-06,6.37147e-05]  Shape=Cylinder  ShapeDims=[1 1]  ShapeUnits=m  ShapeUse=false  Density=1  DensityUnits=kg/m^3  DensityUse=false  GraphicsMode=GFXFILE  GraphicsFileName=RHex1v3_Z - lab_rogz1v1-2.STL  BodyColorSelMode=COLORPALETTE  BodyColor=[0;0.498039;0]  AttachedToCS=CS1  CG=Right$CG$[-0.013584 -0.172621 0.0516204]$WORLD$WORLD$m$[-1 0 0;0 0 1;0 1 0]$3x3 Transform$rad$WORLD$false$lab_rogz1v1-2::CG(AUTOGEN)  WorkingFrames=Right$CS1$[0.00141603 -0.139051 0.00353831]$WORLD$WORLD$m$[-1 0 0;0 0 1;0 1 0]$3x3 Transform$rad$WORLD$false$lab_rogz1v1-2::CS1(AUTOGEN)#Left$CS2$[-0.040584 -0.154051 0.0691787]$WORLD$WORLD$m$[1 0 0;0 1 0;0 0 1]$3x3 Transform$rad$WORLD$true$Body^RHex1v3-1:-:lab_rogz1v1-2::lab_rogz1v1-2(AUTOGEN)#Right$CS3$[-0.013584 -0.154051 -0.0258213]$WORLD$WORLD$m$[1 0 0;0 1 0;0 0 1]$3x3 Transform$rad$WORLD$true$dummy-2:-:lab_rogz1v1-2::lab_rogz1v1-2(AUTOGEN)  CGPos=[-0.013584 -0.172621 0.0516204]  CGRot=[-1 0 0;0 0 1;0 1 0]  CS0Pos=[]  CS0Rot=[]  CS1Pos=[0.00141603 -0.139051 0.00353831]  CS1Rot=[-1 0 0;0 0 1;0 1 0]  CS2Pos=[-0.040584 -0.154051 0.0691787]  CS2Rot=[1 0 0;0 1 0;0 0 1]  CS3Pos=[-0.013584 -0.154051 -0.0258213]  CS3Rot=[1 0 0;0 1 0;0 0 1]  CS4Pos=[]  CS4Rot=[]  CS5Pos=[]  CS5Rot=[]  CS6Pos=[]  CS6Rot=[]  CS7Pos=[]  CS7Rot=[]  CS8Pos=[]  CS8Rot=[]  CS9Pos=[]  CS9Rot=[]  CS10Pos=[]  CS10Rot=[]  CS11Pos=[]  CS11Rot=[]  CS12Pos=[]  CS12Rot=[]  CS13Pos=[]  CS13Rot=[]  CS14Pos=[]  CS14Rot=[]  CS15Pos=[]  CS15Rot=[]  CS16Pos=[]  CS16Rot=[]  CS17Pos=[]  CS17Rot=[]  CS18Pos=[]  CS18Rot=[]  CS19Pos=[]  CS19Rot=[]  CS20Pos=[]  CS20Rot=[]
  Body : PMIOPort  Port=1  Side=Left
  q : Outport
  wires:
  Ground Contact2/1(Fz) -> Mux2/2
  HipControl/1(u) -> Joint Actuator1/1
  Mux3/1 -> HipControl/2(sensor), Demux/1
  Joint Sensor1/1 -> Mux3/1
  Joint Sensor1/2 -> Mux3/2
  Joint Sensor1/3 -> Mux3/3
  Joint Sensor1/4 -> Mux3/4
  Mux2/1 -> q/1
  Pos/1 -> HipControl/1(ref)
  Demux/1 -> Continuous Angle/1
  Demux/2 -> Mux1/2, Continuous Angle/2
  Continuous Angle/1 -> Mux1/1
  Demux/3 -> Mux1/3
  Demux/4 -> Mux1/4
  Mux1/1 -> Mux2/1
  connections:
  lab_rogz1v1-2/RConn1 -- Ground Contact2/LConn1
  Joint Actuator1/RConn1 -- Revolute4/LConn2
  Joint Sensor1/LConn1 -- Revolute4/RConn2
  Revolute4/RConn1 -- lab_rogz1v1-2/LConn1
  Body/RConn1 -- Revolute4/LConn1

== system RHex1v3_Z_0v1b_PID/Right_Rear ==
  Pos : Inport
  Ground Contact1 : Subsystem  AncestorBlock=Ervin/Ground Contact
  HipControl : Subsystem
  Joint Actuator : mblibv1/Sensors &  Actuators/Joint Actuator  UpdateFromCAD=off  PhysicalDomain=Mechanical  PortType=blob  ActuationStyle=Force  AngleUnits=deg  ArcVelocityUnits=deg/s  ArcAccelerationUnits=deg/s^2  CoordPositionUnits=m  VelocityUnits=m/s  AccelerationUnits=m/s^2  ForceUnits=N  TorqueUnits=N-m  ActiveIO=on  Width=1  DialogClass=MechanicalActuatorBlock  Primitive=R1  ReferenceFrame=Absolute (World)
  Joint Sensor : mblibv1/Sensors &  Actuators/Joint Sensor  UpdateFromCAD=off  PhysicalDomain=Mechanical  PortType=blob  Muxed=off  Pose=off  Angle=on  AngleUnits=deg  ArcVelocity=on  ArcVelocityUnits=deg/s  ArcAcceleration=on  ArcAccelerationUnits=deg/s^2  CoordPosition=on  CoordPositionUnits=m  Velocity=off  VelocityUnits=m/s  Acceleration=off  AccelerationUnits=m/s^2  Quaternion=on  QuaternionDT=off  QuaternionDDT=off  QuaternionUnits=off  OutputVector=[1]  ActiveIO=on  Width=4  DialogClass=MechanicalSensorBlock  Primitive=R1  Force=off  ForceUnits=N  Torque=on  TorqueUnits=N*m  ReferenceFrame=Absolute (World)  ReactionSensedSide=Base  ReactionReferenceFrame=Absolute (World)  ReactionForce=off  ReactionForceUnits=N  ReactionMoment=off  ReactionMomentUnits=N*m
  Mux : Mux  Inputs=2
  Mux1 : Mux
  Revolute3 : mblibv1/Joints/Revolute  LConnTagsString=__newl0|SA1  RConnTagsString=__newr0|SA1  UpdateFromCAD=on  PMImportedID=Body^RHex1v3-1:-:lab_rogz1v1-3  NumSAPorts=2  CutJoint=off  MarkAsCut=off  Primitives=prismatic  PrimitiveProps=R1$World$[1,0,0]$revolute  DialogClass=JointBlock  R1Axis=[1,0,0]
  lab_rogz1v1-3 : mblibv1/Bodies/Body  LConnTagsString=CS3  RConnTagsString=CS2  UpdateFromCAD=on  PMImportedID=lab_rogz1v1-3  DialogClass=MechanicalBodyBlock  Mass=0.0510405  MassUnits=kg  InertiaUnits=kg*m^2  Inertia=[7.74224e-05,-1.05103e-11,2.05656e-12;-1.05103e-11,2.14517e-05,-6.14042e-06;2.05656e-12,-6.14042e-06,6.37147e-05]  Shape=Cylinder  ShapeDims=[1 1]  ShapeUnits=m  ShapeUse=false  Density=1  DensityUnits=kg/m^3  DensityUse=false  GraphicsMode=GFXFILE  GraphicsFileName=RHex1v3_Z - lab_rogz1v1-3.STL  BodyColorSelMode=COLORPALETTE  BodyColor=[0;0.498039;0]  AttachedToCS=CS1  CG=Right$CG$[-0.053584 -0.297621 0.0516204]$WORLD$WORLD$m$[-1 0 0;0 0 1;0 1 0]$3x3 Transform$rad$WORLD$false$lab_rogz1v1-3::CG(AUTOGEN)  WorkingFrames=Right$CS1$[-0.038584 -0.264051 0.00353831]$WORLD$WORLD$m$[-1 0 0;0 0 1;0 1 0]$3x3 Transform$rad$WORLD$false$lab_rogz1v1-3::CS1(AUTOGEN)#Right$CS2$[-0.053584 -0.279051 -0.0258213]$WORLD$WORLD$m$[1 0 0;0 1 0;0 0 1]$3x3 Transform$rad$WORLD$true$dummy-3:-:lab_rogz1v1-3::lab_rogz1v1-3(AUTOGEN)#Left$CS3$[-0.080584 -0.279051 0.0691787]$WORLD$WORLD$m$[1 0 0;0 1 0;0 0 1]$3x3 Transform$rad$WORLD$true$Body^RHex1v3-1:-:lab_rogz1v1-3::lab_rogz1v1-3(AUTOGEN)  CGPos=[-0.053584 -0.297621 0.0516204]  CGRot=[-1 0 0;0 0 1;0 1 0]  CS0Pos=[]  CS0Rot=[]  CS1Pos=[-0.038584 -0.264051 0.00353831]  CS1Rot=[-1 0 0;0 0 1;0 1 0]  CS2Pos=[-0.053584 -0.279051 -0.0258213]  CS2Rot=[1 0 0;0 1 0;0 0 1]  CS3Pos=[-0.080584 -0.279051 0.0691787]  CS3Rot=[1 0 0;0 1 0;0 0 1]  CS4Pos=[]  CS4Rot=[]  CS5Pos=[]  CS5Rot=[]  CS6Pos=[]  CS6Rot=[]  CS7Pos=[]  CS7Rot=[]  CS8Pos=[]  CS8Rot=[]  CS9Pos=[]  CS9Rot=[]  CS10Pos=[]  CS10Rot=[]  CS11Pos=[]  CS11Rot=[]  CS12Pos=[]  CS12Rot=[]  CS13Pos=[]  CS13Rot=[]  CS14Pos=[]  CS14Rot=[]  CS15Pos=[]  CS15Rot=[]  CS16Pos=[]  CS16Rot=[]  CS17Pos=[]  CS17Rot=[]  CS18Pos=[]  CS18Rot=[]  CS19Pos=[]  CS19Rot=[]  CS20Pos=[]  CS20Rot=[]
  Body : PMIOPort  Port=1  Side=Left
  q : Outport
  wires:
  Ground Contact1/1(Penettracion) -> Mux/2
  HipControl/1(u) -> Joint Actuator/1
  Mux1/1 -> Mux/1, HipControl/2(sensor)
  Joint Sensor/1 -> Mux1/1
  Joint Sensor/2 -> Mux1/2
  Joint Sensor/3 -> Mux1/3
  Joint Sensor/4 -> Mux1/4
  Pos/1 -> HipControl/1(ref)
  Mux/1 -> q/1
  connections:
  lab_rogz1v1-3/RConn1 -- Ground Contact1/LConn1
  Joint Actuator/RConn1 -- Revolute3/LConn2
  Joint Sensor/LConn1 -- Revolute3/RConn2
  Revolute3/RConn1 -- lab_rogz1v1-3/LConn1
  Body/RConn1 -- Revolute3/LConn1

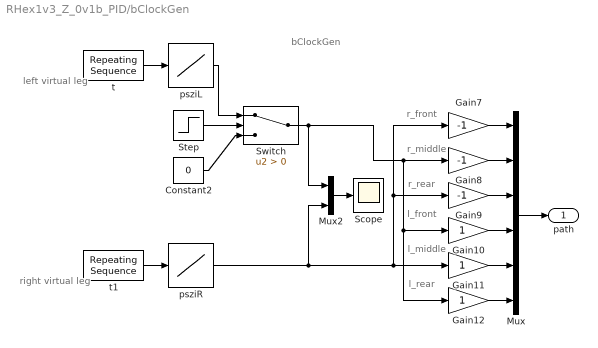
== system RHex1v3_Z_0v1b_PID/bClockGen ==
  note: bClockGen
  note: r_front
  note: r_middle
  note: r_rear
  note: l_front
  note: l_middle
  note: l_rear
  note: left
      | virtual
      | leg
  note: right
      | virtual
      | leg
  Constant2 : Constant  Value=0
  Gain10 : Gain
  Gain11 : Gain
  Gain12 : Gain
  Gain7 : Gain  Gain=-1
  Gain8 : Gain  Gain=-1
  Gain9 : Gain  Gain=-1
  Mux : Mux  Inputs=6
  Mux2 : Mux  Inputs=2
  Scope : Scope
      settings: YMin=0  YMax=350
  Step : Step  Time=tp/2  SampleTime=0
  Switch : Switch  Criteria=u2 > Threshold
  psziL : Lookup_n-D  NumberOfTableDimensions=1  BreakpointsForDimension1=t  Table=psziL  InterpMethod=Cubic spline  ExtrapMethod=Cubic spline  RndMeth=Simplest  InputSameDT=on
  psziR : Lookup_n-D  NumberOfTableDimensions=1  BreakpointsForDimension1=t  Table=psziR  InterpMethod=Cubic spline  ExtrapMethod=Cubic spline  RndMeth=Simplest  InputSameDT=on
  t : simulink/Sources/Repeating Sequence  rep_seq_t=t  rep_seq_y=t
  t1 : simulink/Sources/Repeating Sequence  rep_seq_t=t  rep_seq_y=t
  path : Outport
  wires:
  t1/1 -> psziR/1
  t/1 -> psziL/1
  psziL/1 -> Switch/1
  Mux2/1 -> Scope/1
  Mux/1 -> path/1
  Gain8/1 -> Mux/2
  Switch/1 -> Mux2/1, Gain12/1, Gain10/1, Gain8/1
  Constant2/1 -> Switch/3
  psziR/1 -> Mux2/2, Gain7/1, Gain9/1, Gain11/1
  Step/1 -> Switch/2
  Gain12/1 -> Mux/6
  Gain11/1 -> Mux/5
  Gain10/1 -> Mux/4
  Gain9/1 -> Mux/3
  Gain7/1 -> Mux/1

== system RHex1v3_Z_0v1b_PID/plane ==
  Machine Environment1 : mblibv1/Bodies/Machine Environment  PortType=env  PhysicalDomain=Mechanical  DialogTemplateClass=MECH.MachineEnvironment  SyncWhenCopied=off  Gravity=[0 -9.81 0]  GravityUnits=m/s^2  GravityAsSignal=off  Dimensionality=Auto-detect  AnalysisType=Forward dynamics  LinearAssemblyTolerance=1e-3  LinearAssemblyToleranceUnits=m  AngularAssemblyTolerance=1e-3  AngularAssemblyToleranceUnits=rad  ConstraintSolverType=Stabilizing  ConstraintRelTolerance=1e-4  ConstraintAbsTolerance=1e-4  UseRobustSingularityHandling=off  RedundancyAnalysisToleranceType=Automatically select tolerance  RedundancyAnalysisTolerance=1e-14  StatePerturbationType=Fixed  PerturbationSize=1e-5  VisualizeMachine=on  BodyVisualizationType=Use model default body geometries  BodyColorSelMode=Use model default  DefaultBodyColor=[1 0 0]
  RootGround1 : mblibv1/Bodies/Ground  UpdateFromCAD=on  LeftPortType=env  RightPortType=workingframe  PhysicalDomain=Mechanical  DialogClass=GroundBlock  CoordPosition=[-0.0133749,0.00240505,0.00542379]  CoordPositionUnits=m  StateVectorMgrId=1  MachineId=[1 1]  ShowEnvPort=on
  RootPart1 : mblibv1/Bodies/Body  LConnTagsString=CS3  RConnTagsString=CS2  UpdateFromCAD=on  DialogClass=MechanicalBodyBlock  Mass=0  MassUnits=kg  InertiaUnits=kg*m^2  Inertia=[0,0,0;0,0,0;0,0,0]  Shape=Cylinder  ShapeDims=[1 1]  ShapeUnits=m  ShapeUse=false  Density=1  DensityUnits=kg/m^3  DensityUse=false  GraphicsMode=MACHINE_DEFAULT  BodyColorSelMode=MACHINE_DEFAULT  BodyColor=[1;0;0]  AttachedToCS=CS1  CG=Right$CG$[-0.0133749 0.00240505 0.00542379]$WORLD$WORLD$m$[1 0 0;0 1 0;0 0 1]$3x3 Transform$rad$WORLD$false$none  WorkingFrames=Right$CS1$[0 0 0]$WORLD$WORLD$m$[1 0 0;0 1 0;0 0 1]$3x3 Transform$rad$WORLD$false$none#Right$CS2$[-0.0133749 0.00240505 0.00542379]$WORLD$WORLD$m$[1 0 0;0 1 0;0 0 1]$3x3 Transform$rad$WORLD$true$none#Left$CS3$[-0.0133749 0.00240505 0.00542379]$WORLD$WORLD$m$[1 0 0;0 1 0;0 0 1]$3x3 Transform$rad$WORLD$true$none  CGPos=[-0.0133749 0.00240505 0.00542379]  CGRot=[1 0 0;0 1 0;0 0 1]  CS0Pos=[]  CS0Rot=[]  CS1Pos=[0 0 0]  CS1Rot=[1 0 0;0 1 0;0 0 1]  CS2Pos=[-0.0133749 0.00240505 0.00542379]  CS2Rot=[1 0 0;0 1 0;0 0 1]  CS3Pos=[-0.0133749 0.00240505 0.00542379]  CS3Rot=[1 0 0;0 1 0;0 0 1]  CS4Pos=[]  CS4Rot=[]  CS5Pos=[]  CS5Rot=[]  CS6Pos=[]  CS6Rot=[]  CS7Pos=[]  CS7Rot=[]  CS8Pos=[]  CS8Rot=[]  CS9Pos=[]  CS9Rot=[]  CS10Pos=[]  CS10Rot=[]  CS11Pos=[]  CS11Rot=[]  CS12Pos=[]  CS12Rot=[]  CS13Pos=[]  CS13Rot=[]  CS14Pos=[]  CS14Rot=[]  CS15Pos=[]  CS15Rot=[]  CS16Pos=[]  CS16Rot=[]  CS17Pos=[]  CS17Rot=[]  CS18Pos=[]  CS18Rot=[]  CS19Pos=[]  CS19Rot=[]  CS20Pos=[]  CS20Rot=[]
  Weld : mblibv1/Joints/Weld  LConnTagsString=__newl0  RConnTagsString=__newr0  UpdateFromCAD=on  NumSAPorts=0  CutJoint=off  MarkAsCut=off  Primitives=weld  PrimitiveProps=W$WORLD$[0.57735,0.57735,0.57735]$weld  DialogClass=JointBlock  WAxis=[0.57735,0.57735,0.57735]
  Weld1 : mblibv1/Joints/Weld  LConnTagsString=__newl0  RConnTagsString=__newr0  UpdateFromCAD=on  NumSAPorts=0  CutJoint=off  MarkAsCut=off  Primitives=weld  PrimitiveProps=W$WORLD$[0.57735,0.57735,0.57735]$weld  DialogClass=JointBlock  WAxis=[0.57735,0.57735,0.57735]
  plane-1 : mblibv1/Bodies/Body  LConnTagsString=CS2  UpdateFromCAD=on  DialogClass=MechanicalBodyBlock  Mass=0.25  MassUnits=kg  InertiaUnits=kg*m^2  Inertia=[0.00520835,0,0;0,0.00520835,0;0,0,0.0104167]  Shape=Cylinder  ShapeDims=[1 1]  ShapeUnits=m  ShapeUse=false  Density=1  DensityUnits=kg/m^3  DensityUse=false  GraphicsMode=GFXFILE  GraphicsFileName=Assem1 - plane-1.STL  BodyColorSelMode=COLORPALETTE  BodyColor=[0.792157;0.819608;0.933333]  AttachedToCS=CS1  CG=Right$CG$[-0.0133749 0.00240505 0.00542379]$WORLD$WORLD$m$[1 0 0;0 1 0;0 0 1]$3x3 Transform$rad$WORLD$false$none  WorkingFrames=Right$CS1$[-0.0133749 0.00240505 0.00492379]$WORLD$WORLD$m$[1 0 0;0 1 0;0 0 1]$3x3 Transform$rad$WORLD$false$none#Left$CS2$[-0.0133749 0.00240505 0.00542379]$WORLD$WORLD$m$[1 0 0;0 1 0;0 0 1]$3x3 Transform$rad$WORLD$true$none  CGPos=[-0.0133749 0.00240505 0.00542379]  CGRot=[1 0 0;0 1 0;0 0 1]  CS0Pos=[]  CS0Rot=[]  CS1Pos=[-0.0133749 0.00240505 0.00492379]  CS1Rot=[1 0 0;0 1 0;0 0 1]  CS2Pos=[-0.0133749 0.00240505 0.00542379]  CS2Rot=[1 0 0;0 1 0;0 0 1]  CS3Pos=[]  CS3Rot=[]  CS4Pos=[]  CS4Rot=[]  CS5Pos=[]  CS5Rot=[]  CS6Pos=[]  CS6Rot=[]  CS7Pos=[]  CS7Rot=[]  CS8Pos=[]  CS8Rot=[]  CS9Pos=[]  CS9Rot=[]  CS10Pos=[]  CS10Rot=[]  CS11Pos=[]  CS11Rot=[]  CS12Pos=[]  CS12Rot=[]  CS13Pos=[]  CS13Rot=[]  CS14Pos=[]  CS14Rot=[]  CS15Pos=[]  CS15Rot=[]  CS16Pos=[]  CS16Rot=[]  CS17Pos=[]  CS17Rot=[]  CS18Pos=[]  CS18Rot=[]  CS19Pos=[]  CS19Rot=[]  CS20Pos=[]  CS20Rot=[]
  connections:
  Machine Environment1/RConn1 -- RootGround1/LConn1
  RootGround1/RConn1 -- Weld1/LConn1
  Weld1/RConn1 -- RootPart1/LConn1
  RootPart1/RConn1 -- Weld/LConn1
  Weld/RConn1 -- plane-1/LConn1

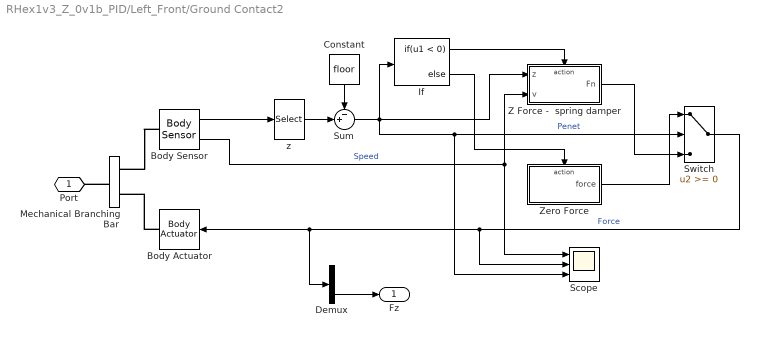
== system RHex1v3_Z_0v1b_PID/Left_Front/Ground Contact2 ==
  Body Actuator : mblibv1/Sensors &  Actuators/Body Actuator  UpdateFromCAD=off  PhysicalDomain=Mechanical  PortType=blob  ActuationStyle=Force  AngleUnits=deg  ArcVelocityUnits=deg/s  ArcAccelerationUnits=deg/s^2  CoordPositionUnits=m  VelocityUnits=m/s  AccelerationUnits=m/s^2  ForceUnits=N  TorqueUnits=N*m  ActiveIO=on  Width=3  DialogClass=MechanicalActuatorBlock  ReferenceFrame=Absolute (World)  Angle=off  CoordPosition=on  Force=on  Torque=off
  Body Sensor : mblibv1/Sensors &  Actuators/Body Sensor  UpdateFromCAD=off  PhysicalDomain=Mechanical  PortType=blob  Muxed=off  Pose=off  Angle=on  AngleUnits=deg  ArcVelocity=off  ArcVelocityUnits=deg/s  ArcAcceleration=off  ArcAccelerationUnits=deg/s^2  CoordPosition=on  CoordPositionUnits=m  Velocity=on  VelocityUnits=m/s  Acceleration=off  AccelerationUnits=m/s^2  Quaternion=on  QuaternionDT=off  QuaternionDDT=off  QuaternionUnits=off  OutputVector=[ 3 3 ]  ActiveIO=on  Width=6  DialogClass=MechanicalSensorBlock  ReferenceFrame=Absolute (World)
  Constant : Constant  Value=floor
  Demux : Demux  Outputs=3
  If : If  IfExpression=u1 < 0
  Mechanical Branching Bar : mblibv1/Utilities/Mechanical Branching Bar  LConnTagsString=_newl0  RConnTagsString=SA0|SA1  UpdateFromCAD=off  DialogClass=MechanicalBranchingBarBlock  NumSAPorts=2
  Scope : Scope  NumInputPorts=3
      settings: YMin=-0.11~-15~-0.025  YMax=0.02~27.5~0.015
  Sum : Sum  Inputs=-+|  SaturateOnIntegerOverflow=on
  Switch : Switch
  Z Force -  spring damper : Subsystem  TreatAsAtomicUnit=on  mask{K=K, C=C, nux=nux, nuy=nuy}
  Zero Force : Subsystem  TreatAsAtomicUnit=on
  z : Selector  InputPortWidth=3  IndexOptions=Index vector (dialog)  Indices=[3]  OutputSizes=1
  Port : PMIOPort  Port=1  Side=Left
  Fz : Outport
  wires:
  Z Force -  spring damper/1(Fn) -> Switch/3
  Zero Force/1(force) -> Switch/1
  Constant/1 -> Sum/1
  Sum/1 -> Switch/2, Scope/3, Z Force -  spring damper/1(z), If/1  "Penet"
  z/1 -> Sum/2
  Switch/1 -> Scope/2, Body Actuator/1, Demux/1  "Force"
  If/1 -> Z Force -  spring damper/Action
  If/2 -> Zero Force/Action
  Body Sensor/2 -> Scope/1, Z Force -  spring damper/2(v)  "Speed"
  Body Sensor/1 -> z/1
  Demux/3 -> Fz/1
  connections:
  Mechanical Branching Bar/LConn1 -- Port/RConn1
  Body Actuator/RConn1 -- Mechanical Branching Bar/RConn2
  Body Sensor/LConn1 -- Mechanical Branching Bar/RConn1

== system RHex1v3_Z_0v1b_PID/Left_Front/HipControl ==
  note: TauControl
  ref : Inport
  sensor : Inport  Port=2
  Continuous Angle : mblibv1/Utilities/Continuous Angle  rad=deg  rads=deg/s
  Demux2 : Demux
  Gain2 : Gain  Gain=Gvis
  PID : simulink/Continuous/PID Controller  Controller=PID  TimeDomain=Continuous-time  SampleTime=1  IntegratorMethod=Forward Euler  FilterMethod=Forward Euler  Form=Parallel  P=kp  I=ki  D=kd  N=kn  InitialConditionSource=internal  InitialConditionForIntegrator=0  InitialConditionForFilter=0  ExternalReset=none  LimitOutput=off  UpperSaturationLimit=inf  LowerSaturationLimit=-inf  LinearizeAsGain=off  AntiWindupMode=none  Kb=1  TrackingMode=off  Kt=1  PParamMin=[]  PParamMax=[]  IParamMin=[]  IParamMax=[]  DParamMin=[]  DParamMax=[]  NParamMin=[]  NParamMax=[]  KbParamMin=[]  KbParamMax=[]  KtParamMin=[]  KtParamMax=[]  POutMin=[]  POutMax=[]  IOutMin=[]  IOutMax=[]  DOutMin=[]  DOutMax=[]  NOutMin=[]  NOutMax=[]  KbOutMin=[]  KbOutMax=[]  KtOutMin=[]  KtOutMax=[]  IntegratorOutMin=[]  IntegratorOutMax=[]  FilterOutMin=[]  FilterOutMax=[]  SumOutMin=[]  SumOutMax=[]  SumI1OutMin=[]  SumI1OutMax=[]  SumI2OutMin=[]  SumI2OutMax=[]  SumI3OutMin=[]  SumI3OutMax=[]  SumDOutMin=[]  SumDOutMax=[]  SaturationOutMin=[]  SaturationOutMax=[]  IntegratorContinuousStateAttributes=''  IntegratorStateMustResolveToSignalObject=off  IntegratorRTWStateStorageClass=Auto  FilterContinuousStateAttributes=''  FilterStateMustResolveToSignalObject=off  FilterRTWStateStorageClass=Auto
  Sum1 : Sum  Inputs=|+-
  Sum2 : Sum  Inputs=|+--
  u : Outport
  wires:
  Demux2/1 -> Continuous Angle/1  "theta"
  sensor/1 -> Demux2/1
  PID/1 -> Sum2/1
  Sum2/1 -> u/1  "u"
  ref/1 -> Sum1/1  "referent_signal"
  Demux2/2 -> Gain2/1, Continuous Angle/2  "dtheta"
  Continuous Angle/1 -> Sum1/2  "cont_rot"
  Sum1/1 -> PID/1  "error"
  Gain2/1 -> Sum2/2  "viscous_damping"
